simulink model "Lab1P8"  (R2017b)
settings: Solver=VariableStepAuto  StartTime=0.0  StopTime=3000  RelTol=1e-3
settings Model: Creator=Cx001la  LastModifiedBy=Cx001la

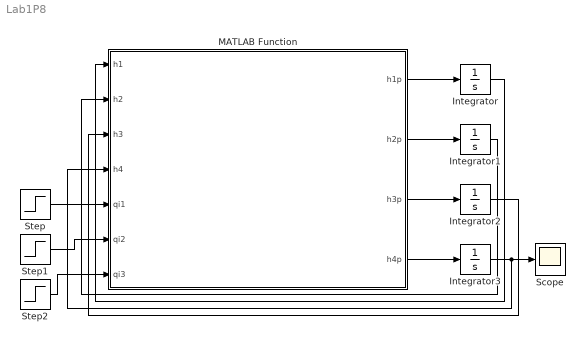
== system Lab1P8 ==
  Integrator{,1..3} (4 alike) : Integrator
  MATLAB Function : MATLAB Function  TreatAsAtomicUnit=on
  Scope : Scope
  Step : Step  SampleTime=0
  Step1 : Step  SampleTime=0
  Step2 : Step  SampleTime=0
  wires:
  MATLAB Function/1(h1p) -> Integrator/1
  MATLAB Function/2(h2p) -> Integrator1/1
  MATLAB Function/3(h3p) -> Integrator2/1
  MATLAB Function/4(h4p) -> Integrator3/1
  Integrator/1 -> MATLAB Function/1(h1)
  Integrator1/1 -> MATLAB Function/2(h2)
  Integrator2/1 -> MATLAB Function/3(h3)
  Integrator3/1 -> Scope/1, MATLAB Function/4(h4)
  Step/1 -> MATLAB Function/5(qi1)
  Step1/1 -> MATLAB Function/6(qi2)
  Step2/1 -> MATLAB Function/7(qi3)

== matlab function Lab1P8/MATLAB Function ==
  data: h1 input; h1p output; h2 input; h3 input; h4 input; qi1 input; qi2 input; qi3 input; h2p output; h3p output; h4p output
function [h1p,h2p,h3p,h4p] = fcn(h1,h2,h3,h4,qi1,qi2,qi3)

R1=10; R2=11; R3=22; R4=50; R5=12; A1=5; A2=8; A3=7; A4=6;
q1=h1/R1;
q2=h1/R2;
q3=h2/R3;
q4=(h3-h4)/R4;
q5=h4/R5;

h1p=(qi1-q1-q2)/A1;
h2p=(qi2-q3)/A2;
h3p=(qi3-q4+q2)/A3;
h4p=(q4-q5+q3)/A4;
